simulink model "HW2_Q.2"  (R2017b)
settings: Solver=VariableStepAuto  StartTime=0.0  StopTime=100  RelTol=1e-3
settings Model: Creator=ali  LastModifiedBy=ali

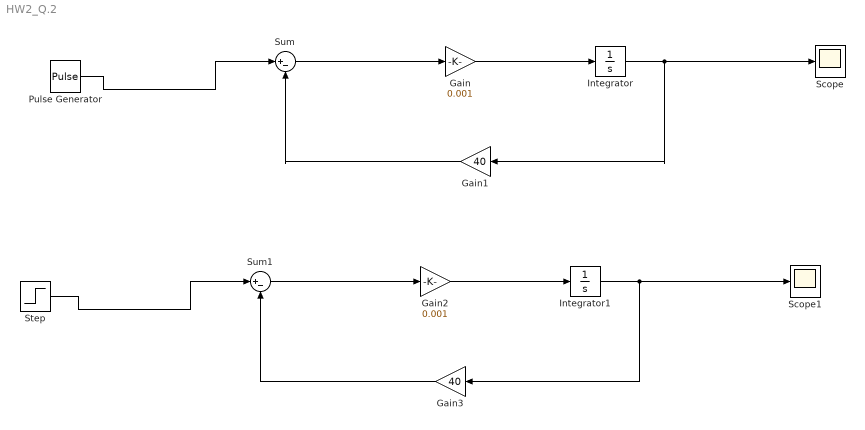
== system HW2_Q.2 ==
  Gain : Gain  Gain=0.001
  Gain1 : Gain  Gain=40
  Gain2 : Gain  Gain=0.001
  Gain3 : Gain  Gain=40
  Integrator : Integrator
  Integrator1 : Integrator
  Pulse Generator : DiscretePulseGenerator  PulseType=Time based  Amplitude=400  Period=100  PulseWidth=10
  Scope : Scope
  Scope1 : Scope
  Step : Step  Time=0  After=500  SampleTime=0
  Sum : Sum  Inputs=|+-
  Sum1 : Sum  Inputs=|+-
  wires:
  Integrator/1 -> Gain1/1, Scope/1
  Sum/1 -> Gain/1
  Gain/1 -> Integrator/1
  Gain1/1 -> Sum/2
  Pulse Generator/1 -> Sum/1
  Integrator1/1 -> Gain3/1, Scope1/1
  Step/1 -> Sum1/1
  Gain3/1 -> Sum1/2
  Sum1/1 -> Gain2/1
  Gain2/1 -> Integrator1/1
